simulink model "Function_Approximation_Ex3"  (R2024a)
settings: Solver=VariableStepAuto  StartTime=0.0  StopTime=512/30e3  RelTol=1e-3
PostLoadFcn:
  | FuncApprox_Init;
InitFcn:
  | FuncApprox_Init;
values from neighbouring files (symbols this model uses):
  max_val = (2^15)-1    (= 32767)    [FuncApprox_Init.m]
  x = ((-N/2):(N/2)-1) / N    [FuncApprox_Init.m]
undefined symbols (not defined in the file or in its folder): S, vsva2197, xcvc1902
libraries: aieDSP x1, aieUtilities x1, vmcUtilities x1
settings Model: Creator=raghug  LastModifiedBy=robg
settings ConfigComp: CovBoundaryAbsTol=1.0e-5

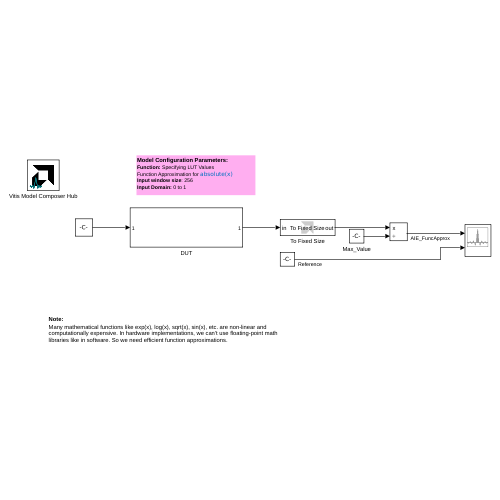
[thumbnail: Simulink's stored preview of the top-level diagram]
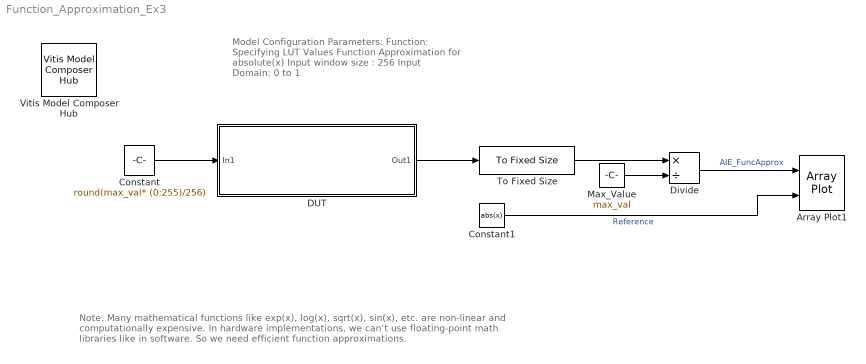
== system Function_Approximation_Ex3 ==
  note: Note:
      | Many mathematical functions like exp(x), log(x), sqrt(x), sin(x), etc. are non-linear and computationally expensive. In hardware implementations, we can’t use floating-point math libraries like in software. So we need efficient function approximations.
  note: Model Configuration Parameters:
      | Function: Specifying LUT Values
      | Function Approximation for absolute(x)
      | Input window size : 256
      | Input Domain: 0 to 1
  Array Plot1 : ArrayPlot  NumInputPorts=2  WindowPosition=[6.000000,33.000000,1920.000000,1127.000000,]  ScopeFrameLocation=window  YLimits=[-0.0625 0.5625]  ShowLegend=on
  Constant : Constant  Value=round(max_val* (0:255)/256)  OutDataTypeStr=int16  SampleTime=1/30e3
  Constant1 : Constant  Value=abs(x)  OutDataTypeStr=single  SampleTime=1/30e3
  DUT : Subsystem
  Divide : Product  Inputs=*/
  Max_Value : Constant  Value=max_val  OutDataTypeStr=single  SampleTime=1/30e3
  To Fixed Size : aieUtilities/To Fixed Size  Mode=Stop simulation when input variable-size signal is not full  OutputSize=Inherit: Same as input  CopyMethod=Buffer samples to form output  HasStatusOutput=on
  Vitis Model Composer Hub : vmcUtilities/Vitis Model Composer Hub  Tag=genX  CodeGeneration=off  StartColumn=1  NumberOfColumns=1  TargetDirectory=./code  exportDesign=off  analyzeDesign=off  validateDesignOnHw=off  ExportType=AI Engines  IpVendor=xilinx.com  IpLibrary=hls  IpVersion=1.0  IpHWLanguage=Verilog  AieCompilerOptions={}  AieSimulatorOptions={}  CreateTestbench=off  TestbenchStackSize=10  RunRtlSim=off  RunCSim=off  RunAieSim=off  AieSimTimeout=50000  RunAieSimProfiling=off  LaunchVitisAnalyzer=off  PlotOutput=off  RunX86Sim=off  X86SimTimeout=10  GenHwImage=off  GenLibadfXo=off  GenHwValidationCode=off  PlatformType=Not Specified  HwSystemType=Baremetal  HwValidationTarget=hw  ProjDevice=xcvc1902-vsva2197-1LP-e-S  ProjDevicePart=xcvc1902-vsva2197-1LP-e-S  AIEType=AIE  SamplePeriod=-1  ClockFrequency=200  DataPathParallelism=1  xilinxfamily=versalaicore  part=xcvc1902  speed=-1LP-e-S  package=vsva2197  directory=./netlist  testbench=off  incr_netlist=off  synthesis_tool=Vivado  clock_wrapper=Clock Enables  dbl_ovrd=According to Block Masks  dcm_input_clock_period=10  sysclk_period=10  simulink_period=1  eval_field=0  LogFileName=''  NThreads=4
  wires:
  Constant/1 -> DUT/1(In1)
  DUT/1(Out1) -> To Fixed Size/1
  To Fixed Size/1 -> Divide/1
  Constant1/1 -> Array Plot1/2  "Reference"
  Divide/1 -> Array Plot1/1  "AIE_FuncApprox"
  Max_Value/1 -> Divide/2

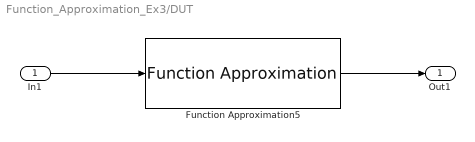
== system Function_Approximation_Ex3/DUT ==
  In1 : Inport
  Function Approximation5 : aieDSP/Function Approximation  AIE_VARIANT=1  data_type=int16  specify_lut_values=<Specify LUT values>  lookup_values=LUTValues  TP_USE_LUT_RELOAD=off  coarse_bits=8  fine_bits=7  domain_mode=0 to 1  num_frames=256  shift_output=0  rnd_mode=Floor  sat_mode=Saturate  blockJsonConstraints=[]  blockJsonConstraintsInternal=[]  spec=vmc_func_approx.json  SerializedMaskParamNames=[]  SerializedMaskParamValues=[]  SerializedMaskParamVisibilities=[]  block_type=Function Approximation  SerializedMaskParamDataypes=uint|typename|typename|data_type|uint|uint|uint|uint|uint|uint|uint|uint  SerializedMaskParamEnumStrArr=0|0|0|0|0|0|0|0 to 1,1 to 2,1 to 4|0|0|Floor,Ceiling,Round to positive infinity,Round to negative infinity,Round symmetrical to infinity,Round symmetrical to zero,Round convergent to even,Round convergent to odd|None,Saturate,Symmetric  SerializedMaskParamEnumValArr=0|0|0|0|0|0|0|0,1,2|0|0|0,1,2,3,4,5,6,7|0,1,3  SerializedMaskParamVectorArr=0|0|0|1|0|0|0|0|0|0|0|0  SerializedMaskParamKeys=AIE_VARIANT|TT_DATA|specify_lut_values|lookup_values|TP_USE_LUT_RELOAD|TP_COARSE_BITS|TP_FINE_BITS|TP_DOMAIN_MODE|TP_WINDOW_VSIZE|TP_SHIFT|TP_RND|TP_SAT
  Out1 : Outport
  wires:
  In1/1 -> Function Approximation5/1
  Function Approximation5/1 -> Out1/1
